simulink model "Decentralized_Cont"  (R2018a)
settings: Solver=VariableStepAuto  StartTime=0.0  StopTime=5  RelTol=1e-3
values from neighbouring files (symbols this model uses):
  Kd_Decent = zeros(7,7)    [ControlSetup.m]
  Kp_Decent = zeros(7,7)    [ControlSetup.m]
libraries: dspinverses x1
(part 1 of 2)
settings Model: Creator=Ricardo  LastModifiedBy=Pedro Ramalho

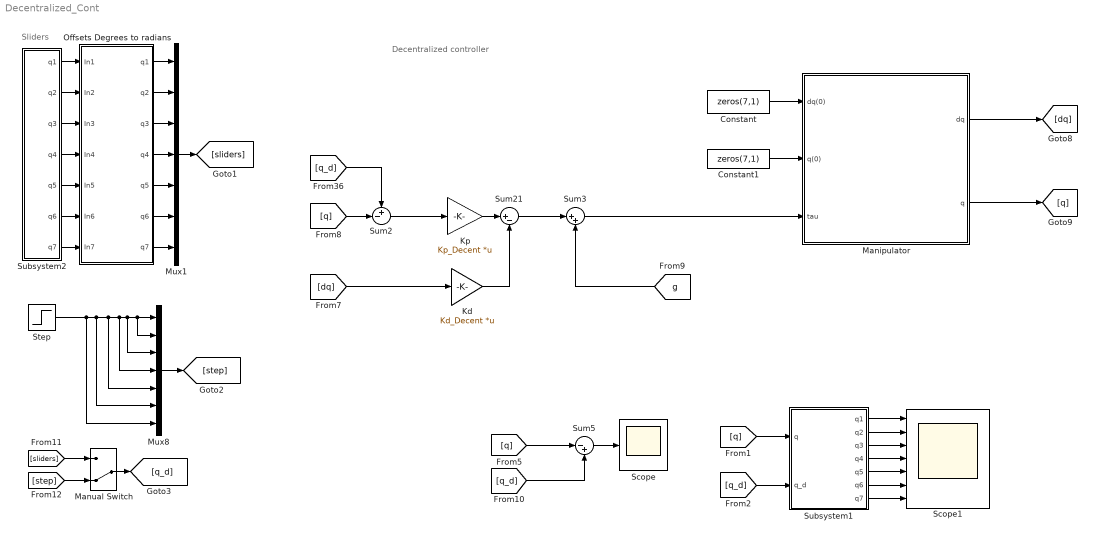
== system Decentralized_Cont ==
  note: Sliders
  note: Decentralized controller
  Constant : Constant  Value=zeros(7,1)
  Constant1 : Constant  Value=zeros(7,1)
  Kd : Gain  Gain=Kd_Decent  Multiplication=Matrix(K*u)
  Kp : Gain  Gain=Kp_Decent  Multiplication=Matrix(K*u)
  Manipulator : Subsystem
  Manual Switch : ManualSwitch  CurrentSetting=0
  Mux1 : Mux  Inputs=7
  Mux8 : Mux  Inputs=7
  Offsets Degrees to radians : Subsystem
  Scope : Scope
  Scope1 : Scope  NumInputPorts=7
  Step : Step  SampleTime=0
  Subsystem1 : Subsystem
  Subsystem2 : Subsystem  mask{q1=1.0, q2=82.800, q3=180.0, q4=-180.0, q5=-180.0, q6=-180.0, q7=180.0}
  Sum2 : Sum  Inputs=+-|
  Sum21 : Sum  Inputs=|+-
  Sum3 : Sum  Inputs=|++
  Sum5 : Sum  Inputs=|-+
  wires:
  Constant1/1 -> Manipulator/2("q(0) ")
  Constant/1 -> Manipulator/1("dq(0) ")
  Sum21/1 -> Sum3/1
  Kp/1 -> Sum21/1
  [g] -> Sum3/2
  [q] -> Sum2/2
  Sum2/1 -> Kp/1
  [dq] -> Kd/1
  Kd/1 -> Sum21/2
  [q_d] -> Sum2/1
  Sum3/1 -> Manipulator/3(tau)
  Manipulator/2(q) -> [q]
  Manipulator/1(dq) -> [dq]
  Manual Switch/1 -> [q_d]
  Offsets Degrees to radians/4(q4) -> Mux1/4
  Offsets Degrees to radians/6(q6) -> Mux1/6
  Offsets Degrees to radians/5(q5) -> Mux1/5
  Offsets Degrees to radians/7(q7) -> Mux1/7
  Offsets Degrees to radians/2(q2) -> Mux1/2
  Mux8/1 -> [step]
  Mux1/1 -> [sliders]
  Subsystem2/7(q7) -> Offsets Degrees to radians/7(In7)
  Subsystem2/2(q2) -> Offsets Degrees to radians/2(In2)
  Subsystem2/6(q6) -> Offsets Degrees to radians/6(In6)
  Subsystem2/3(q3) -> Offsets Degrees to radians/3(In3)
  Offsets Degrees to radians/1(q1) -> Mux1/1
  Offsets Degrees to radians/3(q3) -> Mux1/3
  Subsystem2/1(q1) -> Offsets Degrees to radians/1(In1)
  Step/1 -> Mux8/7, Mux8/6, Mux8/5, Mux8/4, Mux8/1, Mux8/2, Mux8/3
  Subsystem2/4(q4) -> Offsets Degrees to radians/4(In4)
  [step] -> Manual Switch/2
  Subsystem2/5(q5) -> Offsets Degrees to radians/5(In5)
  [sliders] -> Manual Switch/1
  Subsystem1/5(q5) -> Scope1/5
  Subsystem1/4(q4) -> Scope1/4
  Subsystem1/2(q2) -> Scope1/2
  Subsystem1/6(q6) -> Scope1/6
  Subsystem1/3(q3) -> Scope1/3
  [q] -> Subsystem1/1(q)
  Subsystem1/7(q7) -> Scope1/7
  Sum5/1 -> Scope/1
  Subsystem1/1(q1) -> Scope1/1
  [q_d] -> Sum5/2
  [q] -> Sum5/1
  [q_d] -> Subsystem1/2(q_d)

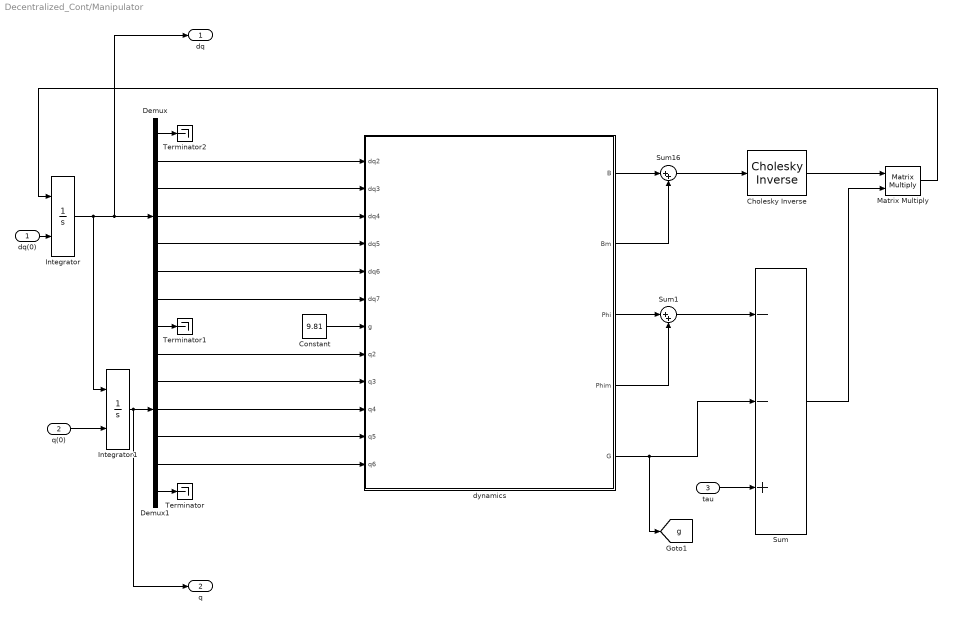
== system Decentralized_Cont/Manipulator ==
  "dq(0) " : Inport
  "q(0) " : Inport  Port=2
  tau : Inport  Port=3
  Cholesky Inverse : dspinverses/Cholesky Inverse  errmode=Warning
      settings: SourceProductName=DSP System Toolbox  SourceProductBaseCode=DS
  Constant : Constant  Value=9.81
  Demux : Demux  Outputs=7
  Demux1 : Demux  Outputs=7
  Integrator : Integrator  InitialConditionSource=external
  Integrator1 : Integrator  InitialConditionSource=external
  Matrix Multiply : Product  Multiplication=Matrix(*)
  Sum : Sum  Inputs=--+
  Sum1 : Sum  Inputs=|++
  Sum16 : Sum  Inputs=|++
  Terminator : Terminator
  Terminator1 : Terminator
  Terminator2 : Terminator
  dynamics : MATLAB Function  TreatAsAtomicUnit=on
  dq : Outport
  q : Outport  Port=2
  tag scope: g=global
  wires:
  Sum1/1 -> Sum/1
  Cholesky Inverse/1 -> Matrix Multiply/1
  dynamics/4(Phim) -> Sum1/2
  dynamics/5(G) -> [g], Sum/2
  Integrator/1 -> dq/1, Demux/1, Integrator1/1
  dynamics/1(B) -> Sum16/1
  "dq(0) "/1 -> Integrator/2
  dynamics/2(Bm) -> Sum16/2
  Sum/1 -> Matrix Multiply/2
  Demux1/5 -> dynamics/11(q5)
  Sum16/1 -> Cholesky Inverse/1
  "q(0) "/1 -> Integrator1/2
  dynamics/3(Phi) -> Sum1/1
  Demux1/1 -> Terminator1/1
  Integrator1/1 -> q/1, Demux1/1
  Demux/6 -> dynamics/5(dq6)
  Demux1/4 -> dynamics/10(q4)
  Constant/1 -> dynamics/7(g)
  Demux/2 -> dynamics/1(dq2)
  Demux/3 -> dynamics/2(dq3)
  Demux/4 -> dynamics/3(dq4)
  Demux/5 -> dynamics/4(dq5)
  Demux/7 -> dynamics/6(dq7)
  Matrix Multiply/1 -> Integrator/1
  tau/1 -> Sum/3
  Demux1/6 -> dynamics/12(q6)
  Demux1/2 -> dynamics/8(q2)
  Demux/1 -> Terminator2/1
  Demux1/3 -> dynamics/9(q3)
  Demux1/7 -> Terminator/1

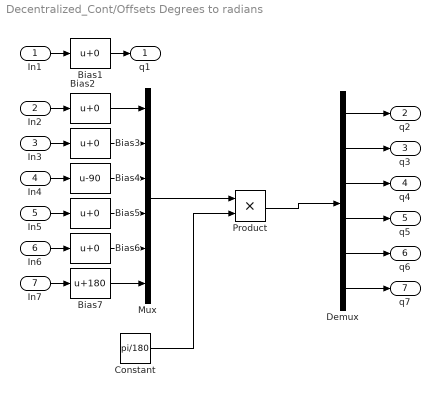
== system Decentralized_Cont/Offsets Degrees to radians ==
  In1 : Inport
  In2 : Inport  Port=2
  In3 : Inport  Port=3
  In4 : Inport  Port=4
  In5 : Inport  Port=5
  In6 : Inport  Port=6
  In7 : Inport  Port=7
  Bias{1..3,5..6} (5 alike) : Bias
  Bias4 : Bias  Bias=-90
  Bias7 : Bias  Bias=180
  Constant : Constant  Value=pi/180
  Demux : Demux  Outputs=6
  Mux : Mux  Inputs=6
  Product : Product
  q1 : Outport
  q2 : Outport  Port=2
  q3 : Outport  Port=3
  q4 : Outport  Port=4
  q5 : Outport  Port=5
  q6 : Outport  Port=6
  q7 : Outport  Port=7
  wires:
  In6/1 -> Bias6/1
  In5/1 -> Bias5/1
  In3/1 -> Bias3/1
  In1/1 -> Bias1/1
  Bias1/1 -> q1/1
  In7/1 -> Bias7/1
  In4/1 -> Bias4/1
  In2/1 -> Bias2/1
  Bias7/1 -> Mux/6
  Bias2/1 -> Mux/1
  Bias3/1 -> Mux/2
  Bias4/1 -> Mux/3
  Bias5/1 -> Mux/4
  Bias6/1 -> Mux/5
  Mux/1 -> Product/1
  Constant/1 -> Product/2
  Demux/1 -> q2/1
  Demux/2 -> q3/1
  Demux/3 -> q4/1
  Demux/4 -> q5/1
  Demux/5 -> q6/1
  Demux/6 -> q7/1
  Product/1 -> Demux/1

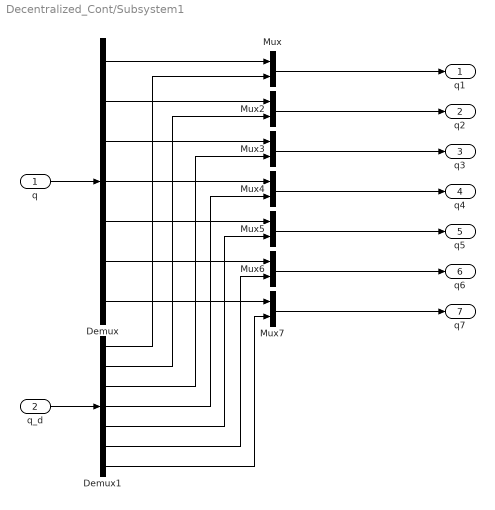
== system Decentralized_Cont/Subsystem1 ==
  q : Inport
  q_d : Inport  Port=2
  Demux : Demux  Outputs=7
  Demux1 : Demux  Outputs=7
  Mux{,2..7} (7 alike) : Mux  Inputs=2
  q1 : Outport
  q2 : Outport  Port=2
  q3 : Outport  Port=3
  q4 : Outport  Port=4
  q5 : Outport  Port=5
  q6 : Outport  Port=6
  q7 : Outport  Port=7
  wires:
  Demux/3 -> Mux3/1
  Demux/7 -> Mux7/1
  Demux1/6 -> Mux6/2
  Demux1/1 -> Mux/2
  Demux/4 -> Mux4/1
  Demux1/4 -> Mux4/2
  Demux/1 -> Mux/1
  Demux1/5 -> Mux5/2
  Mux4/1 -> q4/1
  Demux1/3 -> Mux3/2
  Demux/2 -> Mux2/1
  Demux1/7 -> Mux7/2
  Demux1/2 -> Mux2/2
  Demux/5 -> Mux5/1
  Demux/6 -> Mux6/1
  Mux6/1 -> q6/1
  q/1 -> Demux/1
  Mux/1 -> q1/1
  Mux3/1 -> q3/1
  Mux2/1 -> q2/1
  Mux5/1 -> q5/1
  Mux7/1 -> q7/1
  q_d/1 -> Demux1/1

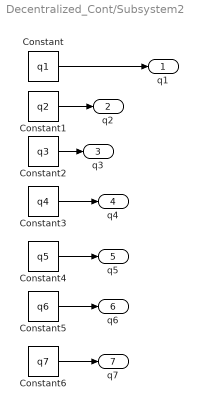
== system Decentralized_Cont/Subsystem2 ==
  Constant : Constant  Value=q1
  Constant1 : Constant  Value=q2
  Constant2 : Constant  Value=q3
  Constant3 : Constant  Value=q4
  Constant4 : Constant  Value=q5
  Constant5 : Constant  Value=q6
  Constant6 : Constant  Value=q7
  q1 : Outport
  q2 : Outport  Port=2
  q3 : Outport  Port=3
  q4 : Outport  Port=4
  q5 : Outport  Port=5
  q6 : Outport  Port=6
  q7 : Outport  Port=7
  wires:
  Constant/1 -> q1/1
  Constant2/1 -> q3/1
  Constant1/1 -> q2/1
  Constant3/1 -> q4/1
  Constant4/1 -> q5/1
  Constant5/1 -> q6/1
  Constant6/1 -> q7/1
